simulink model "task12_8"  (R2021a)
settings: Solver=VariableStepAuto  StartTime=0.0  StopTime=10.0  RelTol=1e-3
settings Model: Creator=reemb  LastModifiedBy=reemb

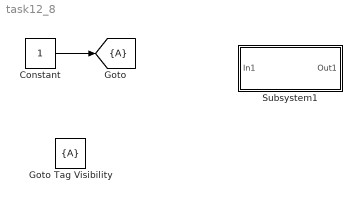
== system task12_8 ==
  Constant : Constant
  Goto Tag Visibility : GotoTagVisibility
  Subsystem1 : Subsystem
  tag scope: A=scoped
  wires:
  Constant/1 -> [A]

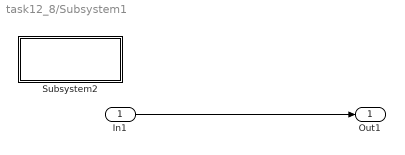
== system task12_8/Subsystem1 ==
  In1 : Inport
  Subsystem2 : Subsystem
  Out1 : Outport
  wires:
  In1/1 -> Out1/1

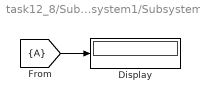
== system task12_8/Subsystem1/Subsystem2 ==
  Display : Display
  wires:
  [A] -> Display/1
